simulink model "Prep"  (R2022a)
settings: Solver=FixedStepAuto  StartTime=0.0  StopTime=100.0  FixedStep=1e-3  RelTol=1e-3  EnableMultiTasking=on
undefined symbols (not defined in the file): D10, D11, D12, D13, D3, D4, D6, D7, D8, D9, PTA0, PTA1, PTB23, PTC2, PTC3, PTC4, PTD0, PTD1, PTD2, PTD3
libraries: frdmk64flib x17
settings Model: ExtModeTrigDuration=5  Creator=ethan  LastModifiedBy=ethan
settings OptimizationCC: EnhancedBackFolding=on  PassReuseOutputArgsAs=Individual arguments  ZeroExternalMemoryAtStartup=off  ZeroInternalMemoryAtStartup=off  MaxStackSize=64  OptimizeBlockOrder=speed  DifferentSizesBufferReuse=on  OptimizationCustomize=off  EfficientTunableParamExpr=on
settings DebuggingCC: ParameterTunabilityLossMsg=error
settings HardwareCC: ProdBitPerPointer=32  ProdBitPerSizeT=32  ProdBitPerPtrDiffT=32  ProdLargestAtomicInteger=Long  ProdLargestAtomicFloat=Double  ProdWordSize=32  ProdHWDeviceType=ARM Compatible->ARM Cortex
settings SFSimCC: MATLABDynamicMemAlloc=off
settings RTWCC: SystemTargetFile=ert.tlc  HardwareBoard=NXP FRDM-K64F  TLCOptions="-aInlineSetEventsForThisBaseRateFcn=TLC_FALSE -aSuppressMultiTaskScheduler=TLC_FALSE  -aRateBasedStepFcn=0"  TemplateMakefile=ert_default_tmf  Toolchain=GNU Tools for ARM Embedded Processors
settings CodeAppCC: ForceParamTrailComments=on  IgnoreCustomStorageClasses=off  OperatorAnnotations=on  SimulinkDataObjDesc=on  SFDataObjDesc=on  InsertBlockDesc=on
settings ERTTargetCC: ExtModeTransport=4  ExtModeMexFile=sendToCommService

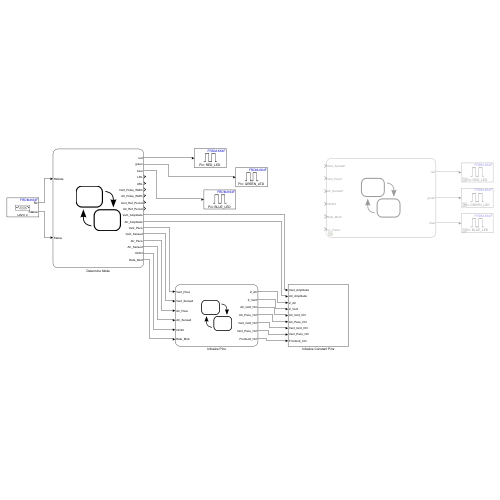
[thumbnail: Simulink's stored preview of the top-level diagram]
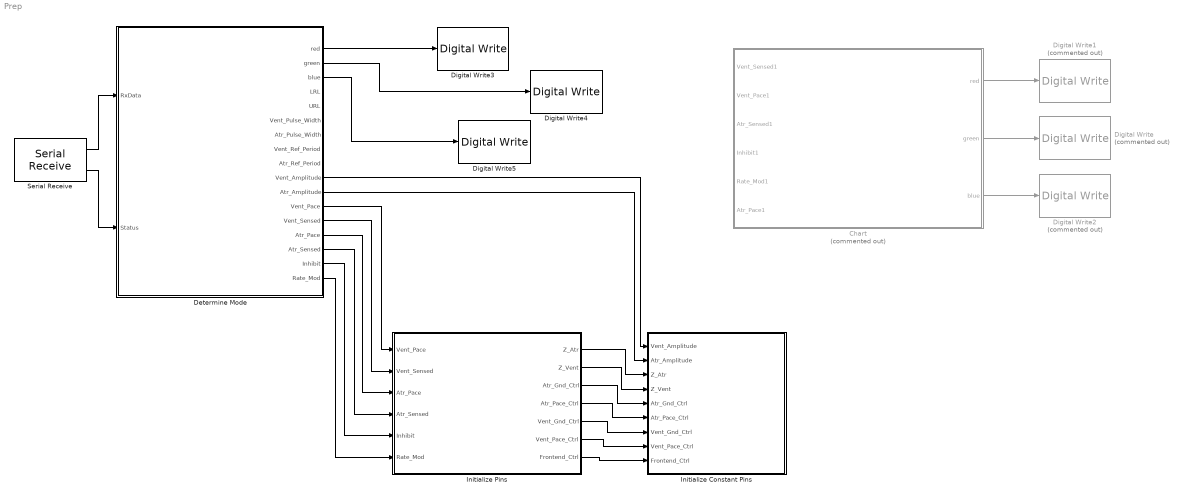
== system Prep ==
  Chart : Stateflow chart  Commented=on  TreatAsAtomicUnit=on
      settings: PortSchema="{\"entries\":[{\"content\":{\"sides\":[{\"content\":{\"connectorIds\":[\"In3\",\"In2\",\"In1\",\"In4\",\"In5\",\"In6\"]},\"type\":\"ConnectorPlacement.EquallySpacedRectSide\",\"uuid\":\"0e4b22a6-a47f-4214-b9ef-749a080df669\"},{\"content\":{\"connectorIds\":[\"Out1\",\"Out2\",\"Out3\"],\"side\":\"RIGHT\"},\"type\":\"ConnectorPlacement.EquallySpacedRectSide\",\"uuid\":\"0adee417-9e0f-4a8f-be57-ef0b3565890b\"},{\"content\":{\"connectorIds\":[],\"side\":\"TOP\"},\"type\":\"ConnectorPlacement.EquallySpacedRectSide\",\"uuid\":\"f4ea0623-47ca-44fd-bb6d-ac8b66ac28ce\"}]},\"type\":\"ConnectorPlacement.EquallySpacedConnector\",\"uuid\":\"8a4551a5-a122-4803-af91-716cc7109805\"}],\"packageUris\":[\"http://schema.mathworks.com/mf0/Connector/R2020b\"],\"version\":\"1.0\"}"
  Determine Mode : Stateflow chart  TreatAsAtomicUnit=on
      settings: PortSchema="{\"entries\":[{\"content\":{\"sides\":[{\"content\":{\"connectorIds\":[\"In1\",\"In2\"]},\"type\":\"ConnectorPlacement.EquallySpacedRectSide\",\"uuid\":\"d3a0267d-6aa2-456b-a992-b2b3c1e06367\"},{\"content\":{\"connectorIds\":[\"Out1\",\"Out2\",\"Out3\",\"Out12\",\"Out5\",\"Out6\",\"Out7\",\"Out10\",\"Out11\",\"Out8\",\"Out9\",\"Out4\",\"Out13\",\"Out14\",\"Out15\",\"Out16\",\"Out17\"],\"side\":\"RIGHT\"},\"type\":\"ConnectorPlacement.EquallySpacedRectSide\",\"uuid\":\"0ed1bc39-4919-47dc-8308-642421d14d88\"},{\"content\":{\"connectorIds\":[],\"side\":\"TOP\"},\"type\":\"ConnectorPlacement.EquallySpacedRectSide\",\"uuid\":\"b0180289-739d-40bc-b384-d64f07ec28c1\"}]},\"type\":\"ConnectorPlacement.EquallySpacedConnector\",\"uuid\":\"4a619b6a-8cfb-4e9f-a229-732ef11ba1d1\"}],\"packageUris\":[\"http://schema.mathworks.com/mf0/Connector/R2020b\"],\"version\":\"1.0\"}"
  Digital Write : frdmk64flib/Digital Write  Commented=on  Whichpin=GREEN_LED
  Digital Write1 : frdmk64flib/Digital Write  Commented=on  Whichpin=RED_LED
  Digital Write2 : frdmk64flib/Digital Write  Commented=on  Whichpin=BLUE_LED
  Digital Write3 : frdmk64flib/Digital Write  Whichpin=RED_LED
  Digital Write4 : frdmk64flib/Digital Write  Whichpin=GREEN_LED
  Digital Write5 : frdmk64flib/Digital Write  Whichpin=BLUE_LED
  Initialize Constant Pins : Subsystem
  Initialize Pins : Stateflow chart  TreatAsAtomicUnit=on
      settings: PortSchema="{\"entries\":[{\"content\":{\"sides\":[{\"content\":{\"connectorIds\":[\"In5\",\"In1\",\"In2\",\"In3\",\"In4\",\"In6\"]},\"type\":\"ConnectorPlacement.EquallySpacedRectSide\",\"uuid\":\"c51a1d0e-b06b-442a-95c0-1a3d5253c08f\"},{\"content\":{\"connectorIds\":[\"Out1\",\"Out2\",\"Out3\",\"Out4\",\"Out5\",\"Out6\",\"Out7\"],\"side\":\"RIGHT\"},\"type\":\"ConnectorPlacement.EquallySpacedRectSide\",\"uuid\":\"41317748-07b9-4449-a7f8-cbb7fdf91266\"},{\"content\":{\"connectorIds\":[],\"side\":\"TOP\"},\"type\":\"ConnectorPlacement.EquallySpacedRectSide\",\"uuid\":\"323f0d8e-b807-4341-a5ce-575c699330d3\"}]},\"type\":\"ConnectorPlacement.EquallySpacedConnector\",\"uuid\":\"143b2e55-0dbd-4f26-ad6f-54df5b80f1ea\"}],\"packageUris\":[\"http://schema.mathworks.com/mf0/Connector/R2020b\"],\"version\":\"1.0\"}"
  Serial Receive : frdmk64flib/Serial Receive  SCIModule=0  Baudrate=uint32(9600)  Parity=None  StopBits=1  HardwareFlowControl=None  ByteOrder=LittleEndian  DataType=int8  DataLength=12  BlockingMode=off  OutputStatus=on  SampleTime=-1
  wires:
  Serial Receive/1 -> Determine Mode/1(RxData)
  Serial Receive/2 -> Determine Mode/2(Status)
  Determine Mode/4(Vent_Pace) -> Initialize Pins/5(Vent_Pace)
  Determine Mode/13(Vent_Sensed) -> Initialize Pins/1(Vent_Sensed)
  Determine Mode/14(Atr_Pace) -> Initialize Pins/2(Atr_Pace)
  Determine Mode/15(Atr_Sensed) -> Initialize Pins/3(Atr_Sensed)
  Determine Mode/16(Inhibit) -> Initialize Pins/4(Inhibit)
  Determine Mode/17(Rate_Mod) -> Initialize Pins/6(Rate_Mod)
  Initialize Pins/6(Vent_Pace_Ctrl) -> Initialize Constant Pins/8(Vent_Pace_Ctrl)
  Initialize Pins/1(Z_Atr) -> Initialize Constant Pins/3(Z_Atr)
  Initialize Pins/5(Vent_Gnd_Ctrl) -> Initialize Constant Pins/7(Vent_Gnd_Ctrl)
  Initialize Pins/2(Z_Vent) -> Initialize Constant Pins/4(Z_Vent)
  Initialize Pins/4(Atr_Pace_Ctrl) -> Initialize Constant Pins/6(Atr_Pace_Ctrl)
  Initialize Pins/3(Atr_Gnd_Ctrl) -> Initialize Constant Pins/5(Atr_Gnd_Ctrl)
  Initialize Pins/7(Frontend_Ctrl) -> Initialize Constant Pins/9(Frontend_Ctrl)
  Determine Mode/8(Vent_Amplitude) -> Initialize Constant Pins/1(Vent_Amplitude)
  Determine Mode/9(Atr_Amplitude) -> Initialize Constant Pins/2(Atr_Amplitude)
  Chart/1(red) -> Digital Write1/1
  Chart/3(blue) -> Digital Write2/1
  Chart/2(green) -> Digital Write/1
  Determine Mode/1(red) -> Digital Write3/1
  Determine Mode/2(green) -> Digital Write4/1
  Determine Mode/3(blue) -> Digital Write5/1

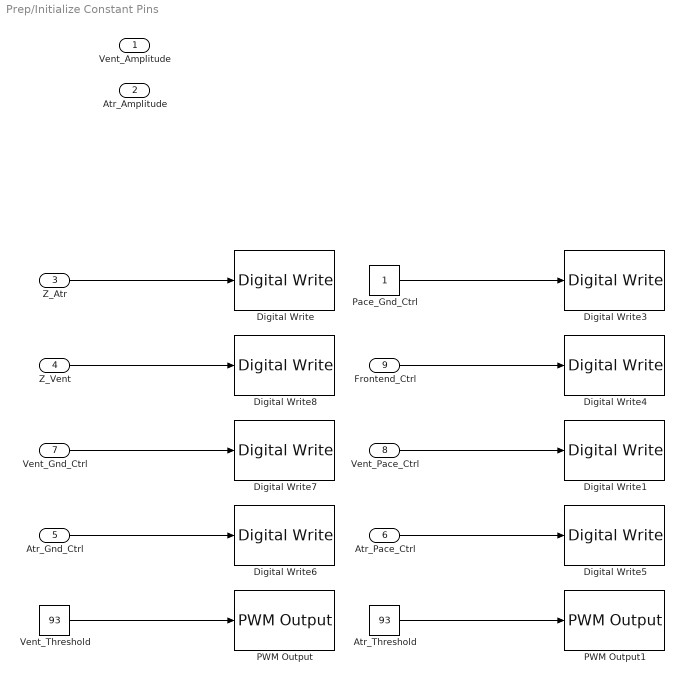
== system Prep/Initialize Constant Pins ==
  Vent_Amplitude : Inport
  Atr_Amplitude : Inport  Port=2
  Z_Atr : Inport  Port=3
  Z_Vent : Inport  Port=4
  Atr_Gnd_Ctrl : Inport  Port=5
  Atr_Pace_Ctrl : Inport  Port=6
  Vent_Gnd_Ctrl : Inport  Port=7
  Vent_Pace_Ctrl : Inport  Port=8
  Frontend_Ctrl : Inport  Port=9
  Atr_Threshold : Constant  Value=93  OutDataTypeStr=int8
  Digital Write : frdmk64flib/Digital Write  Whichpin=PTB23 (D4)
  Digital Write1 : frdmk64flib/Digital Write  Whichpin=PTC4 (D9)
  Digital Write3 : frdmk64flib/Digital Write  Whichpin=PTD0 (D10)
  Digital Write4 : frdmk64flib/Digital Write  Whichpin=PTD1 (D13)
  Digital Write5 : frdmk64flib/Digital Write  Whichpin=PTA0 (D8)
  Digital Write6 : frdmk64flib/Digital Write  Whichpin=PTD2 (D11)
  Digital Write7 : frdmk64flib/Digital Write  Whichpin=PTD3 (D12)
  Digital Write8 : frdmk64flib/Digital Write  Whichpin=PTC3 (D7)
  PWM Output : frdmk64flib/PWM Output  Whichpin=PTA1 (D3)  InitialFrequency=2000  InitialDutyCycle=0
  PWM Output1 : frdmk64flib/PWM Output  Whichpin=PTC2 (D6)  InitialFrequency=2000  InitialDutyCycle=0
  Pace_Gnd_Ctrl : Constant  SampleTime=-1
  Vent_Threshold : Constant  Value=93  OutDataTypeStr=int8
  wires:
  Z_Atr/1 -> Digital Write/1
  Vent_Pace_Ctrl/1 -> Digital Write1/1
  Z_Vent/1 -> Digital Write8/1
  Atr_Gnd_Ctrl/1 -> Digital Write6/1
  Vent_Gnd_Ctrl/1 -> Digital Write7/1
  Atr_Pace_Ctrl/1 -> Digital Write5/1
  Frontend_Ctrl/1 -> Digital Write4/1
  Vent_Threshold/1 -> PWM Output/1
  Atr_Threshold/1 -> PWM Output1/1
  Pace_Gnd_Ctrl/1 -> Digital Write3/1

== stateflow chart Prep/Initialize Pins ==
  state Pacing_Ventricle
    entry:
    Atr_Gnd_Ctrl = false;
    Atr_Pace_Ctrl = false;
  state Sensing
    entry:
    Frontend_Ctrl = true;
  state Initialize_Constant_Pins
    entry:
    Z_Atr = false;
    Z_Vent = false;
  state Pacing_Atrium
    entry:
    Vent_Gnd_Ctrl = false;
    Vent_Pace_Ctrl = false;
  (default) -> Initialize_Constant_Pins
  Initialize_Constant_Pins -> Pacing_Ventricle [order 1] : [Vent_Pace == 1]
  Pacing_Ventricle -> Sensing : [Inhibit == 1]
  Pacing_Atrium -> Sensing : [Inhibit == 1]
  Initialize_Constant_Pins -> Pacing_Atrium [order 2] : [Atr_Pace ==1]
  data: Z_Atr output; Z_Vent output; Atr_Gnd_Ctrl output; Atr_Pace_Ctrl output; Vent_Gnd_Ctrl output; Vent_Sensed input; Atr_Pace input; Atr_Sensed input; Inhibit input; Vent_Pace input; Rate_Mod input; Vent_Pace_Ctrl output; Frontend_Ctrl output

== stateflow chart Prep/Chart ==
  state VOO
    entry:
    red = true;
  state Initialize_All_Variables
    entry:
    Vent_Pace = Vent_Pace1;
    Vent_Sensed = Vent_Sensed1;
    Atr_Pace = Atr_Pace1;
    Atr_Sensed = Atr_Sensed1;
    Inhibit = Inhibit1;
    Rate_Mod = Rate_Mod1;
  state VVI
    entry:
    blue = true;
    after(500,msec)
    blue = false;
  state VOOR
    entry:
    red = true;
    after(500,msec)
    red = false;
    after(500,msec)
    red = true;
    after(500,msec)
    red = false;
  state VVIR
    entry:
    blue = true;
    after(500,msec)
    blue = false;
    after(500,msec)
    blue = true;
    after(500,msec)
    blue = false;
  state AOO
    entry:
    green = true;
    after(500,msec)
    green = false;
  state AOOR
    entry:
    green = true;
    after(500,msec)
    green = false;
    after(500,msec)
    green = true;
    after(500,msec)
    green = false;
  state AAI
    entry:
    green = true;
    after(500,msec)
    green = false;
    after(500,msec)
    red = true;
    after(500,msec)
    red = false
  state AAIR
    entry:
    green = true;
    after(500,msec)
    green = false;
    after(500,msec)
    blue = true;
    after(500,msec)
    blue = false;
  (default) -> Initialize_All_Variables
  (junction 24) -> VOO [order 1] : [Rate_Mod == 0]
  (junction 24) -> VOOR [order 2] : [Rate_Mod == 1]
  (junction 15) -> (junction 24) [order 1] : [Vent_Sensed == 0]
  Initialize_All_Variables -> (junction 15) [order 1] : [Vent_Pace == 1 && Atr_Pace == 0]
  (junction 15) -> (junction 36) [order 2] : [Vent_Sensed == 1 && Inhibit == 1]
  (junction 36) -> VVI [order 1] : [Rate_Mod == 0]
  Initialize_All_Variables -> (junction 50) [order 2] : [Vent_Pace == 0 && Atr_Pace == 1]
  (junction 36) -> VVIR [order 2] : [Rate_Mod == 1]
  (junction 51) -> AOO [order 1] : [Rate_Mod == 0]
  (junction 50) -> (junction 51) [order 1] : [Atr_Sensed == 1]
  (junction 51) -> AOOR [order 2] : [Rate_Mod == 1]
  (junction 50) -> (junction 39) [order 2] : [Atr_Sensed == 1 && Inhibit == 1]
  (junction 39) -> AAI [order 1] : [Rate_Mod == 0]
  (junction 39) -> AAIR [order 2] : [Rate_Mod == 1]
  data: Atr_Sensed1 input; Vent_Pace1 input; Vent_Sensed1 input; Inhibit1 input; Rate_Mod1 input; red output; green output; blue output; Vent_Pace local; Vent_Sensed local; Atr_Pace local; Atr_Sensed local; Inhibit local; Rate_Mod local; Atr_Pace1 input

== stateflow chart Prep/Determine Mode ==
  settings: executeAtInitialization=1
  state Sense_Ventrical
    entry:
    Vent_Sensed = 1;
    Inhibit = 1;
  state Pace_Ventricle
    entry:
    Vent_Pace = 1;
  state No_Sensing
  state Input_Parameters
    entry:
    LRL = RxData(5);
    URL = RxData(6);
    Vent_Pulse_Width = RxData(7);
    Atr_Pulse_Width = RxData(8);
    Vent_Amplitude = RxData(9);
    Atr_Amplitude = RxData(10);
    Vent_Ref_Period = RxData(11);
    Atr_Ref_Period = RxData(12);
  state Initialize_Variables
    entry:
    Vent_Pace = 0;
    Atr_Pace = 0;
    Vent_Sensed = 0;
    Atr_Sensed = 0;
    Inhibit = 0;
    Rate_Mod = 0;
    red = false;
    green = false;
    blue = false;
  state Rate_Modulation
    entry:
    Rate_Mod = 1;
  state Pace_Atrium
    entry:
    Atr_Pace = 1;
  state Sense_Atrium
    entry:
    Atr_Sensed = 1;
    Inhibit = 1;
  state Wait_For_Data
  state Dual_Pacing
    entry:
    Vent_Pace =1;
    Atr_Pace = 1;
  state Dual_Sensing
    entry:
    Vent_Sensed =1;
    Atr_Sensed = 1;
  state green
    entry:
    green = true;
  state red
    entry:
    red = true;
  state blue
    entry:
    blue = true;
  state all_off
    entry:
    red = false;
    green = false;
    blue = false;
  Pace_Ventricle -> Sense_Ventrical [order 1] : [RxData(3) == hex2dec('30')]
  Sense_Ventrical -> Rate_Modulation [order 1] : [RxData(4) == hex2dec('40')]
  Sense_Ventrical -> Input_Parameters [order 2] : [RxData(4) == hex2dec('43')]
  Pace_Ventricle -> No_Sensing [order 2] : [RxData(3) == hex2dec('32')]
  No_Sensing -> Input_Parameters [order 2] : [RxData(4) == hex2dec('43')]
  (junction 25) -> Pace_Ventricle [order 1] : [RxData(2) == hex2dec('15')]
  Pace_Ventricle -> green [order 3]
  Pace_Atrium -> No_Sensing [order 2] : [RxData(3) == hex2dec('32')]
  No_Sensing -> Rate_Modulation [order 1] : [RxData(4) == hex2dec('40')]
  (default) -> Initialize_Variables
  (junction 18) -> Wait_For_Data [order 2]
  Rate_Modulation -> Input_Parameters
  Sense_Atrium -> Rate_Modulation [order 1] : [RxData(4) == hex2dec('40')]
  Initialize_Variables -> Wait_For_Data
  Wait_For_Data -> (junction 18) : [Status == 0]
  (junction 18) -> (junction 25) [order 1] : [RxData(1) == hex2dec('10')]
  (junction 25) -> Pace_Atrium [order 3] : [RxData(2) == hex2dec('20')]
  Dual_Sensing -> Rate_Modulation [order 1] : [RxData(4) == hex2dec('40')]
  Pace_Atrium -> Sense_Atrium [order 1] : [RxData(3) == hex2dec('34')]
  (junction 25) -> Dual_Pacing [order 2] : [RxData(2) == hex2dec('25')]
  Sense_Atrium -> Input_Parameters [order 2] : [RxData(4) == hex2dec('43')]
  Pace_Atrium -> blue [order 3]
  Dual_Sensing -> Input_Parameters [order 2] : [RxData(4) == hex2dec('43')]
  Input_Parameters -> Initialize_Variables
  Dual_Pacing -> Dual_Sensing [order 1] : [RxData(3) == hex2dec('36')]
  all_off -> Initialize_Variables
  Dual_Pacing -> red [order 2]
  green -> all_off : after(500,msec)
  red -> all_off : after(500,msec)
  blue -> all_off : after(500,msec)
  data: red output; green output; blue output; RxData input; Status input; Vent_Pace output; URL output; Vent_Pulse_Width output; Atr_Pulse_Width output; Vent_Amplitude output; Atr_Amplitude output; Vent_Ref_Period output; Atr_Ref_Period output; LRL output; Vent_Sensed output; Atr_Pace output; Atr_Sensed output; Inhibit output; Rate_Mod output
